simulink model "example1"  (Simulink 7.3)
settings: Solver=FixedStepDiscrete  StartTime=0.0  StopTime=10  FixedStep=0.02  RelTol=1e-3
libraries: voderiv x6, simulink x1
settings Model: Creator=badania  LastModifiedBy=dominik
settings DebuggingCC: StrictBusMsg=ErrorLevel1

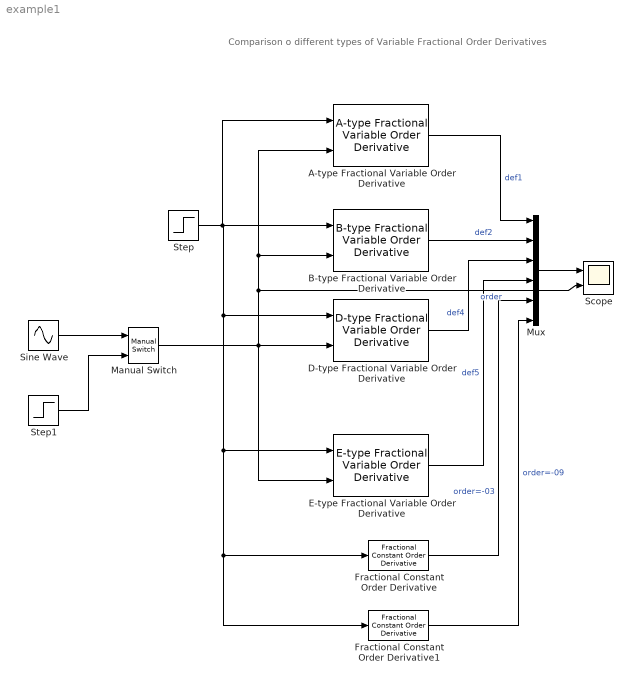
== system example1 ==
  note: Comparison o different types of Variable Fractional Order Derivatives
  A-type Fractional Variable Order Derivative : voderiv/A-type Fractional Variable Order Derivative  N=1  Nbuf=500  Ts=0.02
  B-type Fractional Variable Order Derivative : voderiv/B-type Fractional Variable Order Derivative  N=1  Nbuf=500  Ts=0.02
  D-type Fractional Variable Order Derivative : voderiv/D-type Fractional Variable Order Derivative  N=1  Nbuf=500  Ts=0.02
  E-type Fractional Variable Order Derivative : voderiv/E-type Fractional Variable Order Derivative  N=1  Nbuf=500  Ts=0.02
  Fractional Constant Order Derivative : voderiv/Fractional Constant Order Derivative  N=-0.3  Nbuf=500  Ts=0.02
  Fractional Constant Order Derivative1 : voderiv/Fractional Constant Order Derivative  N=-0.9  Nbuf=500  Ts=0.02
  Manual Switch : simulink/Signal Routing/Manual Switch  SystemSampleTime=-1  sw=0  action=0  varsize=off
  Mux : Mux  Inputs=6
  Scope : Scope  NumInputPorts=2
      settings: TickLabels=on  YMin=-5~-5  YMax=5~5
  Sine Wave : Sin  Amplitude=0.3  Bias=-0.6  Frequency=1  Phase=0  Samples=10  SampleTime=0.02  Offset=0
  Step : Step  Time=0  SampleTime=0.02
  Step1 : Step  Time=5  Before=-0.3  After=-0.9  SampleTime=0.02
  wires:
  Step/1 -> Fractional Constant Order Derivative/1, Fractional Constant Order Derivative1/1, E-type Fractional Variable Order Derivative/1, D-type Fractional Variable Order Derivative/1, A-type Fractional Variable Order Derivative/1, B-type Fractional Variable Order Derivative/1
  A-type Fractional Variable Order Derivative/1 -> Mux/1  "def1"
  B-type Fractional Variable Order Derivative/1 -> Mux/2  "def2"
  Mux/1 -> Scope/1
  D-type Fractional Variable Order Derivative/1 -> Mux/3  "def4"
  E-type Fractional Variable Order Derivative/1 -> Mux/4  "def5"
  Fractional Constant Order Derivative/1 -> Mux/5  "order=-03"
  Fractional Constant Order Derivative1/1 -> Mux/6  "order=-09"
  Manual Switch/1 -> A-type Fractional Variable Order Derivative/2, B-type Fractional Variable Order Derivative/2, Scope/2, D-type Fractional Variable Order Derivative/2, E-type Fractional Variable Order Derivative/2  "order"
  Sine Wave/1 -> Manual Switch/1
  Step1/1 -> Manual Switch/2
